simulink model "L8T1_HysteresisControlH_BridgeInverter"  (R2021a)
settings: Solver=VariableStepAuto  StartTime=0.0  StopTime=0.05  RelTol=1e-3
libraries: spsIGBTDiodeLib x4, spsVoltageMeasurementLib x2, spsACVoltageSourceLib x1, spsCurrentMeasurementLib x1, spsDCVoltageSourceLib x1, spsSeriesRLCBranchLib x1, spspowerguiLib x1
settings Model: Creator=hp  LastModifiedBy=User

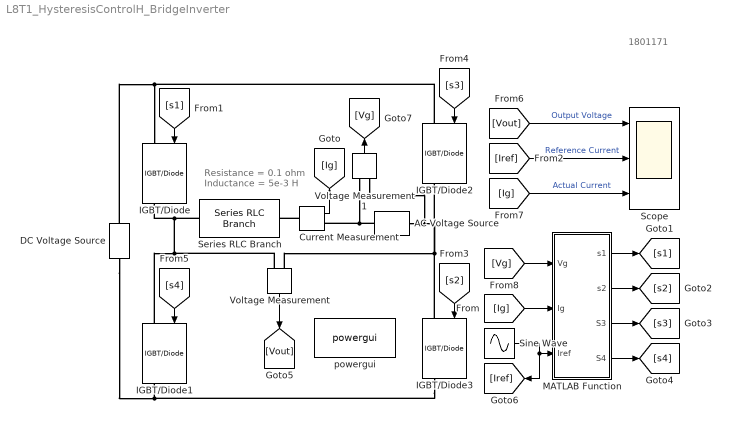
== system L8T1_HysteresisControlH_BridgeInverter ==
  note: Resistance = 0.1 ohm
      | Inductance = 5e-3 H
  note: 1801171
  AC Voltage Source : spsACVoltageSourceLib/AC Voltage Source  Amplitude=220  Phase=0  Frequency=50  SampleTime=0  Measurements=None  BusType=swing  Pref=10e3  Qref=0  Qmin=-inf  Qmax=+inf
  Current Measurement : spsCurrentMeasurementLib/Current Measurement  PhasorSimulation=off  OutputType=Complex  PSBequivalent=0
  DC Voltage Source : spsDCVoltageSourceLib/DC Voltage Source  Amplitude=400  Measurements=None
  IGBT/Diode{,1..3} (4 alike) : spsIGBTDiodeLib/IGBT//Diode  Ron=1e-3  Rs=1e5  Cs=inf  Measurements=on
  MATLAB Function : MATLAB Function  TreatAsAtomicUnit=on
  Scope : Scope  NumInputPorts=3
  Series RLC Branch : spsSeriesRLCBranchLib/Series RLC Branch  LConnTagsString=__new0  RConnTagsString=__new0  BranchType=RL  Resistance=0.1  Inductance=5e-3  SetiL0=off  InitialCurrent=0  Capacitance=1e-6  Setx0=off  InitialVoltage=0  Measurements=None
  Sine Wave : Sin  Amplitude=20  Frequency=2*3.1416*50  SampleTime=0
  Voltage Measurement : spsVoltageMeasurementLib/Voltage Measurement  PhasorSimulation=off  OutputType=Complex  PSBequivalent=0
  Voltage Measurement1 : spsVoltageMeasurementLib/Voltage Measurement  PhasorSimulation=off  OutputType=Complex  PSBequivalent=0
  powergui : spspowerguiLib/powergui  Priority=1  SimulationMode=Discrete  SampleTime=50e-6  frequency=60  Iterations=50  frequencyindice=50  Pbase=100e6  ErrMax=1e-4  UnitsV=kV  UnitsW=MW  buscounter=0  FunctionMessages=off  echomessages=off  EnableUseOfTLC=off  CurrentSourceSwitches=off  DisableSnubberDevices=off  DisableRonSwitches=off  DisableVfSwitches=off  DisplayEquations=off  AutomaticDiscreteSolvers=off  SolverType=Tustin/Backward Euler (TBE)  Interpol=off  ExternalGateDelay=off  methode=off  Ts=100  x0status=blocks  SPID=on  SwTol=0  HookPort=off  NonlinearTolerance=1e-4  nMaxIteration=100  ContinueOnMaxIteration=off  RestoreLinks=warning  ResistiveCurrentMeasurement=off  Frange=[0:2:500]  Ylog=off  Xlog=on  ShowGrid=off  save=off  variable=ZData  structure=0  ZoomFFT=off  StartTime=0.0  cycles=1  DisplayStyle=1  fundamental=60  FreqAxis=off  MaxFrequency=1000  frequencyindicesteady=1  RmsSteady=1  display=off
  wires:
  Current Measurement/1 -> [Ig]
  [Ig] -> MATLAB Function/2(Ig)
  Sine Wave/1 -> [Iref], MATLAB Function/3(Iref)
  MATLAB Function/1(s1) -> [s1]
  MATLAB Function/2(s2) -> [s2]
  MATLAB Function/3(S3) -> [s3]
  MATLAB Function/4(S4) -> [s4]
  [s1] -> IGBT/Diode/1
  [s2] -> IGBT/Diode3/1
  [s3] -> IGBT/Diode2/1
  [s4] -> IGBT/Diode1/1
  [Vout] -> Scope/1  "Output Voltage"
  Voltage Measurement/1 -> [Vout]
  [Iref] -> Scope/2  "Reference Current"
  [Ig] -> Scope/3  "Actual Current"
  Voltage Measurement1/1 -> [Vg]
  [Vg] -> MATLAB Function/1(Vg)
  connections:
  IGBT/Diode1/LConn1 -- Series RLC Branch/LConn1 -- IGBT/Diode/RConn1 -- Voltage Measurement/LConn1
  DC Voltage Source/RConn1 -- IGBT/Diode2/LConn1 -- IGBT/Diode/LConn1
  DC Voltage Source/LConn1 -- IGBT/Diode3/RConn1 -- IGBT/Diode1/RConn1
  IGBT/Diode3/LConn1 -- Voltage Measurement/LConn2 -- Voltage Measurement1/LConn2 -- AC Voltage Source/LConn1 -- IGBT/Diode2/RConn1
  Current Measurement/LConn1 -- Series RLC Branch/RConn1
  AC Voltage Source/RConn1 -- Voltage Measurement1/LConn1 -- Current Measurement/RConn1

== matlab function L8T1_HysteresisControlH_BridgeInverter/MATLAB Function ==
  data: Vg input; Ig input; s1 output; Iref input; s2 output; S3 output; S4 output
function [s1,s2,S3,S4] = fcn(Vg,Ig,Iref)
persistent Q1;
if isempty(Q1)    Q1=0; end
persistent Q2;
if isempty(Q2)    Q2=0; end
persistent Q3;
if isempty(Q3)    Q3=0; end
persistent Q4;
if isempty(Q4)    Q4=0; end
delta=1;
e=Ig-Iref;
if Vg>=0
    if e<=-delta
        Q1=1;   Q2=1;   Q3=0;   Q4=0;
    elseif e>=delta
        Q1=1;   Q2=0;   Q3=1;   Q4=0;
    else 
        Q1=Q1;  Q2=Q2;  Q3=Q3;  Q4=Q4;
    end
else
    if e<=-delta
        Q1=1;   Q2=0;   Q3=1;   Q4=0;
    elseif e>=delta
        Q1=0;   Q2=0;   Q3=1;   Q4=1;
    else
        Q1=Q1;  Q2=Q2;  Q3=Q3;  Q4=Q4;
    end
   end
   s1=Q1;   s2=Q2;   S3=Q3;   S4=Q4;
end
